simulink model "case6"  (R2024b)
settings: Solver=FixedStepAuto  StartTime=0  StopTime=1  FixedStep=1e-7  RelTol=1e-3
values from neighbouring files (symbols this model uses):
  SG_D_1_D = 0.01056    [IEEE9_case_parameters.m]    (also in case1_parameters.m; case2_parameters.m; case3_parameters.m; case4_parameters.m)
  SG_D_1_EnableSaturation = 0    [IEEE9_case_parameters.m]    (also in case1_parameters.m; case2_parameters.m; case3_parameters.m; case4_parameters.m)
  SG_D_1_f0 = 60    [IEEE9_case_parameters.m]    (also in case1_parameters.m; case2_parameters.m; case3_parameters.m; case4_parameters.m)
  SG_D_1_H = 7.5    [IEEE9_case_parameters.m]    (also in case1_parameters.m; case2_parameters.m; case3_parameters.m; case4_parameters.m)
  SG_D_1_K_A = 20    [IEEE9_case_parameters.m]    (also in case1_parameters.m; case2_parameters.m; case3_parameters.m; case4_parameters.m)
  SG_D_1_K_E = 1.000000e+1    (= 10)    [IEEE9_case_parameters.m]    (also in case1_parameters.m; case2_parameters.m; case3_parameters.m; case4_parameters.m)
  SG_D_1_K_F = 2.363    [IEEE9_case_parameters.m]    (also in case1_parameters.m; case2_parameters.m; case3_parameters.m; case4_parameters.m)
  SG_D_1_K_s = 0.5    [IEEE9_case_parameters.m]    (also in case1_parameters.m = 5; case2_parameters.m = 5; case3_parameters.m = 5; case4_parameters.m = 5)
  SG_D_1_R_a = 0.001088    [IEEE9_case_parameters.m]    (also in case1_parameters.m; case2_parameters.m; case3_parameters.m; case4_parameters.m)
  SG_D_1_S_A = 1    [IEEE9_case_parameters.m]    (also in case1_parameters.m; case2_parameters.m; case3_parameters.m; case4_parameters.m)
  SG_D_1_S_B = 0.103    [IEEE9_case_parameters.m]    (also in case1_parameters.m; case2_parameters.m; case3_parameters.m; case4_parameters.m)
  SG_D_1_S_N = 10.659857    [IEEE9_case_parameters.m]    (also in case1_parameters.m; case2_parameters.m; case3_parameters.m; case4_parameters.m)
  SG_D_1_SpeedPara = 200    [IEEE9_case_parameters.m]    (also in case1_parameters.m; case2_parameters.m; case3_parameters.m; case4_parameters.m)
  SG_D_1_T_0 = 0.720173    [IEEE9_case_parameters.m]    (also in case1_parameters.m = 0.755522; case2_parameters.m = 0.808931; case3_parameters.m = 0.869402; case4_parameters.m = 0.729316)
  SG_D_1_T_1 = 0.3    [IEEE9_case_parameters.m]    (also in case1_parameters.m; case2_parameters.m; case3_parameters.m; case4_parameters.m)
  SG_D_1_T_2 = 0.05    [IEEE9_case_parameters.m]    (also in case1_parameters.m; case2_parameters.m; case3_parameters.m; case4_parameters.m)
  SG_D_1_T_3 = 0.02    [IEEE9_case_parameters.m]    (also in case1_parameters.m; case2_parameters.m; case3_parameters.m; case4_parameters.m)
  SG_D_1_T_4 = 0.005    [IEEE9_case_parameters.m]    (also in case1_parameters.m; case2_parameters.m; case3_parameters.m; case4_parameters.m)
  SG_D_1_T_A = 0.02    [IEEE9_case_parameters.m]    (also in case1_parameters.m; case2_parameters.m; case3_parameters.m; case4_parameters.m)
  SG_D_1_T_dd = 8.000000e+0    (= 8)    [IEEE9_case_parameters.m]    (also in case1_parameters.m; case2_parameters.m; case3_parameters.m; case4_parameters.m)
  SG_D_1_T_ddd = 0.04    [IEEE9_case_parameters.m]    (also in case1_parameters.m; case2_parameters.m; case3_parameters.m; case4_parameters.m)
  SG_D_1_T_E = 0.314    [IEEE9_case_parameters.m]    (also in case1_parameters.m; case2_parameters.m; case3_parameters.m; case4_parameters.m)
  SG_D_1_T_F = 0.35    [IEEE9_case_parameters.m]    (also in case1_parameters.m; case2_parameters.m; case3_parameters.m; case4_parameters.m)
  SG_D_1_T_qd = 0.8    [IEEE9_case_parameters.m]    (also in case1_parameters.m; case2_parameters.m; case3_parameters.m; case4_parameters.m)
  SG_D_1_T_qdd = 0.02    [IEEE9_case_parameters.m]    (also in case1_parameters.m; case2_parameters.m; case3_parameters.m; case4_parameters.m)
  SG_D_1_T_speed = 0.1    [IEEE9_case_parameters.m]    (also in case1_parameters.m = 200; case2_parameters.m = 200; case3_parameters.m = 200; case4_parameters.m = 200)
  SG_D_1_T_w = 0.5    [IEEE9_case_parameters.m]    (also in case1_parameters.m; case2_parameters.m; case3_parameters.m; case4_parameters.m)
  SG_D_1_V_ref = 1.990276    [IEEE9_case_parameters.m]    (also in case1_parameters.m = 2.042296; case2_parameters.m = 2.051388; case3_parameters.m = 2.089584; case4_parameters.m = 2.01845)
  SG_D_1_w_ref = 376.991118    [IEEE9_case_parameters.m]    (also in case1_parameters.m; case2_parameters.m; case3_parameters.m; case4_parameters.m)
  SG_D_1_wb = 6.000000e+1    (= 60)    [IEEE9_case_parameters.m]    (also in case1_parameters.m; case2_parameters.m; case3_parameters.m; case4_parameters.m)
  SG_D_1_x_d = 1.9    [IEEE9_case_parameters.m]    (also in case1_parameters.m; case2_parameters.m; case3_parameters.m; case4_parameters.m)
  SG_D_1_x_dd = 0.302    [IEEE9_case_parameters.m]    (also in case1_parameters.m; case2_parameters.m; case3_parameters.m; case4_parameters.m)
  SG_D_1_x_ddd = 0.204    [IEEE9_case_parameters.m]    (also in case1_parameters.m; case2_parameters.m; case3_parameters.m; case4_parameters.m)
  SG_D_1_x_l = 0.05    [IEEE9_case_parameters.m]    (also in case1_parameters.m; case2_parameters.m; case3_parameters.m; case4_parameters.m)
  SG_D_1_x_q = 1.3    [IEEE9_case_parameters.m]    (also in case1_parameters.m; case2_parameters.m; case3_parameters.m; case4_parameters.m)
  SG_D_1_x_qd = 0.5    [IEEE9_case_parameters.m]    (also in case1_parameters.m; case2_parameters.m; case3_parameters.m; case4_parameters.m)
  SG_D_1_x_qdd = 0.3    [IEEE9_case_parameters.m]    (also in case1_parameters.m; case2_parameters.m; case3_parameters.m; case4_parameters.m)
  SG_D_2_D = 0.02    [IEEE9_case_parameters.m]    (also in case1_parameters.m; case2_parameters.m; case3_parameters.m; case4_parameters.m)
  SG_D_2_EnableSaturation = 0    [IEEE9_case_parameters.m]    (also in case1_parameters.m; case2_parameters.m; case3_parameters.m; case4_parameters.m)
  SG_D_2_f0 = 60    [IEEE9_case_parameters.m]    (also in case1_parameters.m; case2_parameters.m; case3_parameters.m; case4_parameters.m)
  SG_D_2_H = 8.000000e+0    (= 8)    [IEEE9_case_parameters.m]    (also in case1_parameters.m; case2_parameters.m; case3_parameters.m; case4_parameters.m)
  SG_D_2_K_A = 20    [IEEE9_case_parameters.m]    (also in case1_parameters.m; case2_parameters.m; case3_parameters.m; case4_parameters.m)
  SG_D_2_K_E = 1.000000e+1    (= 10)    [IEEE9_case_parameters.m]    (also in case1_parameters.m; case2_parameters.m; case3_parameters.m; case4_parameters.m)
  SG_D_2_K_F = 2.363    [IEEE9_case_parameters.m]    (also in case1_parameters.m; case2_parameters.m; case3_parameters.m; case4_parameters.m)
  SG_D_2_K_s = 0.5    [IEEE9_case_parameters.m]    (also in case1_parameters.m = 4; case2_parameters.m = 4; case3_parameters.m = 4; case4_parameters.m = 4)
  SG_D_2_R_a = 0.001088    [IEEE9_case_parameters.m]    (also in case1_parameters.m; case2_parameters.m; case3_parameters.m; case4_parameters.m)
  SG_D_2_S_A = 1    [IEEE9_case_parameters.m]    (also in case1_parameters.m; case2_parameters.m; case3_parameters.m; case4_parameters.m)
  SG_D_2_S_B = 0.103    [IEEE9_case_parameters.m]    (also in case1_parameters.m; case2_parameters.m; case3_parameters.m; case4_parameters.m)
  SG_D_2_S_N = 10.659857    [IEEE9_case_parameters.m]    (also in case1_parameters.m; case2_parameters.m; case3_parameters.m; case4_parameters.m)
  SG_D_2_SpeedPara = 200    [IEEE9_case_parameters.m]    (also in case1_parameters.m; case2_parameters.m; case3_parameters.m; case4_parameters.m)
  SG_D_2_T_0 = 1.632913    [IEEE9_case_parameters.m]    (also in case1_parameters.m = 1.632925; case2_parameters.m = 1.632915; case3_parameters.m = 1.632914; case4_parameters.m = 1.632927)
  SG_D_2_T_1 = 0.2    [IEEE9_case_parameters.m]    (also in case1_parameters.m; case2_parameters.m; case3_parameters.m; case4_parameters.m)
  SG_D_2_T_2 = 0.05    [IEEE9_case_parameters.m]    (also in case1_parameters.m; case2_parameters.m; case3_parameters.m; case4_parameters.m)
  SG_D_2_T_3 = 0.02    [IEEE9_case_parameters.m]    (also in case1_parameters.m; case2_parameters.m; case3_parameters.m; case4_parameters.m)
  SG_D_2_T_4 = 0.005    [IEEE9_case_parameters.m]    (also in case1_parameters.m; case2_parameters.m; case3_parameters.m; case4_parameters.m)
  SG_D_2_T_A = 0.02    [IEEE9_case_parameters.m]    (also in case1_parameters.m; case2_parameters.m; case3_parameters.m; case4_parameters.m)
  SG_D_2_T_dd = 7.9    [IEEE9_case_parameters.m]    (also in case1_parameters.m; case2_parameters.m; case3_parameters.m; case4_parameters.m)
  SG_D_2_T_ddd = 0.04    [IEEE9_case_parameters.m]    (also in case1_parameters.m; case2_parameters.m; case3_parameters.m; case4_parameters.m)
  SG_D_2_T_E = 0.314    [IEEE9_case_parameters.m]    (also in case1_parameters.m; case2_parameters.m; case3_parameters.m; case4_parameters.m)
  SG_D_2_T_F = 0.35    [IEEE9_case_parameters.m]    (also in case1_parameters.m; case2_parameters.m; case3_parameters.m; case4_parameters.m)
  SG_D_2_T_qd = 0.8    [IEEE9_case_parameters.m]    (also in case1_parameters.m; case2_parameters.m; case3_parameters.m; case4_parameters.m)
  SG_D_2_T_qdd = 0.015    [IEEE9_case_parameters.m]    (also in case1_parameters.m; case2_parameters.m; case3_parameters.m; case4_parameters.m)
  SG_D_2_T_speed = 0.1    [IEEE9_case_parameters.m]    (also in case1_parameters.m = 150; case2_parameters.m = 150; case3_parameters.m = 150; case4_parameters.m = 150)
  SG_D_2_T_w = 0.35    [IEEE9_case_parameters.m]    (also in case1_parameters.m; case2_parameters.m; case3_parameters.m; case4_parameters.m)
  SG_D_2_V_ref = 2.58547    [IEEE9_case_parameters.m]    (also in case1_parameters.m = 2.597896; case2_parameters.m = 2.587136; case3_parameters.m = 2.586042; case4_parameters.m = 2.599679)
  SG_D_2_w_ref = 376.991118    [IEEE9_case_parameters.m]    (also in case1_parameters.m; case2_parameters.m; case3_parameters.m; case4_parameters.m)
  SG_D_2_wb = 6.000000e+1    (= 60)    [IEEE9_case_parameters.m]    (also in case1_parameters.m; case2_parameters.m; case3_parameters.m; case4_parameters.m)
  SG_D_2_x_d = 1.8    [IEEE9_case_parameters.m]    (also in case1_parameters.m; case2_parameters.m; case3_parameters.m; case4_parameters.m)
  SG_D_2_x_dd = 0.302    [IEEE9_case_parameters.m]    (also in case1_parameters.m; case2_parameters.m; case3_parameters.m; case4_parameters.m)
  SG_D_2_x_ddd = 0.204    [IEEE9_case_parameters.m]    (also in case1_parameters.m; case2_parameters.m; case3_parameters.m; case4_parameters.m)
  SG_D_2_x_l = 0.05    [IEEE9_case_parameters.m]    (also in case1_parameters.m; case2_parameters.m; case3_parameters.m; case4_parameters.m)
  SG_D_2_x_q = 1.25    [IEEE9_case_parameters.m]    (also in case1_parameters.m; case2_parameters.m; case3_parameters.m; case4_parameters.m)
  SG_D_2_x_qd = 0.5    [IEEE9_case_parameters.m]    (also in case1_parameters.m; case2_parameters.m; case3_parameters.m; case4_parameters.m)
  SG_D_2_x_qdd = 0.3    [IEEE9_case_parameters.m]    (also in case1_parameters.m; case2_parameters.m; case3_parameters.m; case4_parameters.m)
  SG_D_3_D = 0.02    [IEEE9_case_parameters.m]    (also in case1_parameters.m; case2_parameters.m; case3_parameters.m; case4_parameters.m)
  SG_D_3_EnableSaturation = 0    [IEEE9_case_parameters.m]    (also in case1_parameters.m; case2_parameters.m; case3_parameters.m; case4_parameters.m)
  SG_D_3_f0 = 60    [IEEE9_case_parameters.m]    (also in case1_parameters.m; case2_parameters.m; case3_parameters.m; case4_parameters.m)
  SG_D_3_H = 7.7    [IEEE9_case_parameters.m]    (also in case1_parameters.m; case2_parameters.m; case3_parameters.m; case4_parameters.m)
  SG_D_3_K_A = 20    [IEEE9_case_parameters.m]    (also in case1_parameters.m; case2_parameters.m; case3_parameters.m; case4_parameters.m)
  SG_D_3_K_E = 1.000000e+1    (= 10)    [IEEE9_case_parameters.m]    (also in case1_parameters.m; case2_parameters.m; case3_parameters.m; case4_parameters.m)
  SG_D_3_K_F = 2.363    [IEEE9_case_parameters.m]    (also in case1_parameters.m; case2_parameters.m; case3_parameters.m; case4_parameters.m)
  SG_D_3_K_s = 0.2    [IEEE9_case_parameters.m]    (also in case1_parameters.m = 2; case2_parameters.m = 2; case3_parameters.m = 2; case4_parameters.m = 2)
  SG_D_3_R_a = 0.001088    [IEEE9_case_parameters.m]    (also in case1_parameters.m; case2_parameters.m; case3_parameters.m; case4_parameters.m)
  SG_D_3_S_A = 1    [IEEE9_case_parameters.m]    (also in case1_parameters.m; case2_parameters.m; case3_parameters.m; case4_parameters.m)
  SG_D_3_S_B = 0.103    [IEEE9_case_parameters.m]    (also in case1_parameters.m; case2_parameters.m; case3_parameters.m; case4_parameters.m)
  SG_D_3_S_N = 10.659857    [IEEE9_case_parameters.m]    (also in case1_parameters.m; case2_parameters.m; case3_parameters.m; case4_parameters.m)
  SG_D_3_SpeedPara = 200    [IEEE9_case_parameters.m]    (also in case1_parameters.m; case2_parameters.m; case3_parameters.m; case4_parameters.m)
  SG_D_3_T_0 = 0.850788    [IEEE9_case_parameters.m]    (also in case1_parameters.m = 0.850786; case2_parameters.m = 0.850787; case3_parameters.m; case4_parameters.m = 0.850786)
  SG_D_3_T_1 = 0.2    [IEEE9_case_parameters.m]    (also in case1_parameters.m; case2_parameters.m; case3_parameters.m; case4_parameters.m)
  SG_D_3_T_2 = 0.05    [IEEE9_case_parameters.m]    (also in case1_parameters.m; case2_parameters.m; case3_parameters.m; case4_parameters.m)
  SG_D_3_T_3 = 0.02    [IEEE9_case_parameters.m]    (also in case1_parameters.m; case2_parameters.m; case3_parameters.m; case4_parameters.m)
  SG_D_3_T_4 = 0.005    [IEEE9_case_parameters.m]    (also in case1_parameters.m; case2_parameters.m; case3_parameters.m; case4_parameters.m)
  SG_D_3_T_A = 0.02    [IEEE9_case_parameters.m]    (also in case1_parameters.m; case2_parameters.m; case3_parameters.m; case4_parameters.m)
  SG_D_3_T_dd = 8.1    [IEEE9_case_parameters.m]    (also in case1_parameters.m; case2_parameters.m; case3_parameters.m; case4_parameters.m)
  SG_D_3_T_ddd = 0.04    [IEEE9_case_parameters.m]    (also in case1_parameters.m; case2_parameters.m; case3_parameters.m; case4_parameters.m)
  SG_D_3_T_E = 0.314    [IEEE9_case_parameters.m]    (also in case1_parameters.m; case2_parameters.m; case3_parameters.m; case4_parameters.m)
  SG_D_3_T_F = 0.35    [IEEE9_case_parameters.m]    (also in case1_parameters.m; case2_parameters.m; case3_parameters.m; case4_parameters.m)
  SG_D_3_T_qd = 0.8    [IEEE9_case_parameters.m]    (also in case1_parameters.m; case2_parameters.m; case3_parameters.m; case4_parameters.m)
  SG_D_3_T_qdd = 0.015    [IEEE9_case_parameters.m]    (also in case1_parameters.m; case2_parameters.m; case3_parameters.m; case4_parameters.m)
  SG_D_3_T_speed = 0.1    [IEEE9_case_parameters.m]    (also in case1_parameters.m = 180; case2_parameters.m = 180; case3_parameters.m = 180; case4_parameters.m = 180)
  SG_D_3_T_w = 0.4    [IEEE9_case_parameters.m]    (also in case1_parameters.m; case2_parameters.m; case3_parameters.m; case4_parameters.m)
  SG_D_3_V_ref = 1.892727    [IEEE9_case_parameters.m]    (also in case1_parameters.m = 1.906439; case2_parameters.m = 1.895535; case3_parameters.m = 1.892105; case4_parameters.m = 1.906598)
  SG_D_3_w_ref = 376.991118    [IEEE9_case_parameters.m]    (also in case1_parameters.m; case2_parameters.m; case3_parameters.m; case4_parameters.m)
  SG_D_3_wb = 6.000000e+1    (= 60)    [IEEE9_case_parameters.m]    (also in case1_parameters.m; case2_parameters.m; case3_parameters.m; case4_parameters.m)
  SG_D_3_x_d = 1.85    [IEEE9_case_parameters.m]    (also in case1_parameters.m; case2_parameters.m; case3_parameters.m; case4_parameters.m)
  SG_D_3_x_dd = 0.302    [IEEE9_case_parameters.m]    (also in case1_parameters.m; case2_parameters.m; case3_parameters.m; case4_parameters.m)
  SG_D_3_x_ddd = 0.204    [IEEE9_case_parameters.m]    (also in case1_parameters.m; case2_parameters.m; case3_parameters.m; case4_parameters.m)
  SG_D_3_x_l = 0.05    [IEEE9_case_parameters.m]    (also in case1_parameters.m; case2_parameters.m; case3_parameters.m; case4_parameters.m)
  SG_D_3_x_q = 1.2    [IEEE9_case_parameters.m]    (also in case1_parameters.m; case2_parameters.m; case3_parameters.m; case4_parameters.m)
  SG_D_3_x_qd = 0.5    [IEEE9_case_parameters.m]    (also in case1_parameters.m; case2_parameters.m; case3_parameters.m; case4_parameters.m)
  SG_D_3_x_qdd = 0.3    [IEEE9_case_parameters.m]    (also in case1_parameters.m; case2_parameters.m; case3_parameters.m; case4_parameters.m)
(part 2 of 12)

== system case6/SG_D_2 ==
  v_d_SG_D_2 : Inport
  v_q_SG_D_2 : Inport  Port=2
  E_fd_SG_D_2 : Integrator  InitialCondition=3.1522779272193207
  Px_1_SG_D_2 : Integrator  InitialCondition=0.0
  Px_2_SG_D_2 : Integrator  InitialCondition=0.0
  Px_3_SG_D_2 : Integrator  InitialCondition=-2.786907381010745e-25
  R_f_SG_D_2 : Integrator  InitialCondition=21.28237926291216
  T_e_SG_D_2_block : Subsystem
  T_m_SG_D_2 : Integrator  InitialCondition=1.632905998125784
  V_f_SG_D_2 : Integrator  InitialCondition=31.52277927219321
  d_E_fd_SG_D_2_block : Subsystem
  d_Px_1_SG_D_2_block : Subsystem
  d_Px_2_SG_D_2_block : Subsystem
  d_Px_3_SG_D_2_block : Subsystem
  d_R_f_SG_D_2_block : Subsystem
  d_T_m_SG_D_2_block : Subsystem
  d_V_f_SG_D_2_block : Subsystem
  d_psi_1d_SG_D_2_block : Subsystem
  d_psi_d_SG_D_2_block : Subsystem
  d_psi_fd_SG_D_2_block : Subsystem
  d_psi_gq_SG_D_2_block : Subsystem
  d_psi_kq_SG_D_2_block : Subsystem
  d_psi_q_SG_D_2_block : Subsystem
  d_theta_SG_D_2_block : Subsystem
  d_w_SG_D_2_block : Subsystem
  i_d_SG_D_2_block : Subsystem
  i_q_SG_D_2_block : Subsystem
  psi_1d_SG_D_2 : Integrator  InitialCondition=0.5661877704992511
  psi_d_SG_D_2 : Integrator  InitialCondition=0.49229948030724896
  psi_fd_SG_D_2 : Integrator  InitialCondition=0.9385847530669411
  psi_gq_SG_D_2 : Integrator  InitialCondition=0.523477654580875
  psi_kq_SG_D_2 : Integrator  InitialCondition=-0.8375642473294
  psi_q_SG_D_2 : Integrator  InitialCondition=-0.8724627576347918
  theta_SG_D_2 : Integrator  InitialCondition=1.2302637808215569
  theta_SG_D_2_out_block : Subsystem
  w_SG_D_2 : Integrator  InitialCondition=376.99111843077515
  w_SG_D_2_out_block : Subsystem
  i_d_SG_D_2 : Outport
  i_q_SG_D_2 : Outport  Port=2
  T_e_SG_D_2 : Outport  Port=3
  w_SG_D_2_out : Outport  Port=4
  theta_SG_D_2_out : Outport  Port=5
  wires:
  T_e_SG_D_2_block/1(Blockout_T_e_SG_D_2_2a19a) -> T_e_SG_D_2/1
  d_Px_2_SG_D_2_block/1(Blockout_d_Px_2_SG_D_2_75597) -> Px_2_SG_D_2/1
  d_T_m_SG_D_2_block/1(Blockout_d_T_m_SG_D_2_8c4dc) -> T_m_SG_D_2/1
  w_SG_D_2/1 -> d_psi_d_SG_D_2_block/9(State_w_SG_D_2_32109), d_w_SG_D_2_block/1(State_w_SG_D_2_9540e), d_psi_q_SG_D_2_block/9(State_w_SG_D_2_3c58c), d_V_f_SG_D_2_block/8(State_w_SG_D_2_9ec77), d_V_f_SG_D_2_block/13(State_w_SG_D_2_fc7ef), d_theta_SG_D_2_block/1(State_w_SG_D_2_cb344), d_Px_1_SG_D_2_block/2(State_w_SG_D_2_e2895), d_T_m_SG_D_2_block/1(State_w_SG_D_2_d1516), d_Px_2_SG_D_2_block/4(State_w_SG_D_2_c3292), w_SG_D_2_out_block/1(State_w_SG_D_2_a7da0), d_Px_3_SG_D_2_block/6(State_w_SG_D_2_e2d04)
  psi_q_SG_D_2/1 -> d_psi_d_SG_D_2_block/8(State_psi_q_SG_D_2_e45e5), d_psi_gq_SG_D_2_block/6(State_psi_q_SG_D_2_3086c), d_psi_kq_SG_D_2_block/5(State_psi_q_SG_D_2_b3f78), d_w_SG_D_2_block/6(State_psi_q_SG_D_2_7f967), d_w_SG_D_2_block/7(State_psi_q_SG_D_2_af0e3), d_V_f_SG_D_2_block/11(State_psi_q_SG_D_2_aa693), d_psi_q_SG_D_2_block/3(State_psi_q_SG_D_2_571db), i_d_SG_D_2_block/3(State_psi_q_SG_D_2_46eac), T_e_SG_D_2_block/4(State_psi_q_SG_D_2_aa98c), d_psi_gq_SG_D_2_block/9(State_psi_q_SG_D_2_9e01f), T_e_SG_D_2_block/5(State_psi_q_SG_D_2_0c973), i_q_SG_D_2_block/3(State_psi_q_SG_D_2_e3c89), d_V_f_SG_D_2_block/7(State_psi_q_SG_D_2_f03d5)
  w_SG_D_2_out_block/1(Blockout_w_SG_D_2_out_1bf45) -> w_SG_D_2_out/1
  d_theta_SG_D_2_block/1(Blockout_d_theta_SG_D_2_0f7ec) -> theta_SG_D_2/1
  psi_kq_SG_D_2/1 -> d_psi_q_SG_D_2_block/2(State_psi_kq_SG_D_2_25a64), d_psi_gq_SG_D_2_block/3(State_psi_kq_SG_D_2_00780), d_psi_gq_SG_D_2_block/5(State_psi_kq_SG_D_2_d1b3d), d_psi_kq_SG_D_2_block/2(State_psi_kq_SG_D_2_17791), d_w_SG_D_2_block/5(State_psi_kq_SG_D_2_8152c), d_V_f_SG_D_2_block/10(State_psi_kq_SG_D_2_e2d6f), d_psi_gq_SG_D_2_block/8(State_psi_kq_SG_D_2_4b899), i_d_SG_D_2_block/2(State_psi_kq_SG_D_2_f39d8), d_psi_kq_SG_D_2_block/4(State_psi_kq_SG_D_2_51ab3), i_q_SG_D_2_block/2(State_psi_kq_SG_D_2_930b2), T_e_SG_D_2_block/3(State_psi_kq_SG_D_2_bf31f)
  d_Px_1_SG_D_2_block/1(Blockout_d_Px_1_SG_D_2_cd7c4) -> Px_1_SG_D_2/1
  d_Px_3_SG_D_2_block/1(Blockout_d_Px_3_SG_D_2_4fae6) -> Px_3_SG_D_2/1
  T_m_SG_D_2/1 -> d_T_m_SG_D_2_block/2(State_T_m_SG_D_2_36b08), d_w_SG_D_2_block/2(State_T_m_SG_D_2_05bd7)
  Px_2_SG_D_2/1 -> d_Px_3_SG_D_2_block/2(State_Px_2_SG_D_2_d06b1), d_Px_2_SG_D_2_block/1(State_Px_2_SG_D_2_b5883), d_Px_3_SG_D_2_block/3(State_Px_2_SG_D_2_72320)
  i_d_SG_D_2_block/1(Blockout_i_d_SG_D_2_1c8b0) -> i_d_SG_D_2/1
  psi_d_SG_D_2/1 -> d_psi_fd_SG_D_2_block/6(State_psi_d_SG_D_2_52887), d_psi_fd_SG_D_2_block/9(State_psi_d_SG_D_2_9b3b0), d_psi_d_SG_D_2_block/2(State_psi_d_SG_D_2_1074f), d_psi_q_SG_D_2_block/8(State_psi_d_SG_D_2_57873), d_psi_1d_SG_D_2_block/4(State_psi_d_SG_D_2_2211c), d_w_SG_D_2_block/3(State_psi_d_SG_D_2_9dc7c), d_V_f_SG_D_2_block/5(State_psi_d_SG_D_2_4bbd3), d_V_f_SG_D_2_block/12(State_psi_d_SG_D_2_77c88), i_d_SG_D_2_block/6(State_psi_d_SG_D_2_503d3), T_e_SG_D_2_block/1(State_psi_d_SG_D_2_01b1a), i_q_SG_D_2_block/6(State_psi_d_SG_D_2_f3333), d_w_SG_D_2_block/9(State_psi_d_SG_D_2_75c16), T_e_SG_D_2_block/7(State_psi_d_SG_D_2_d0b7a)
  Px_1_SG_D_2/1 -> d_Px_2_SG_D_2_block/3(State_Px_1_SG_D_2_e0226), d_Px_3_SG_D_2_block/5(State_Px_1_SG_D_2_c353d), d_Px_3_SG_D_2_block/4(State_Px_1_SG_D_2_bdfda), d_Px_1_SG_D_2_block/1(State_Px_1_SG_D_2_84b2f), d_Px_2_SG_D_2_block/2(State_Px_1_SG_D_2_b4148)
  psi_gq_SG_D_2/1 -> d_psi_q_SG_D_2_block/1(State_psi_gq_SG_D_2_12de1), d_psi_gq_SG_D_2_block/1(State_psi_gq_SG_D_2_36994), d_psi_gq_SG_D_2_block/2(State_psi_gq_SG_D_2_8aea1), d_psi_gq_SG_D_2_block/4(State_psi_gq_SG_D_2_0cdbf), d_psi_kq_SG_D_2_block/1(State_psi_gq_SG_D_2_dc43a), d_w_SG_D_2_block/4(State_psi_gq_SG_D_2_1ea7a), d_psi_gq_SG_D_2_block/7(State_psi_gq_SG_D_2_14d3b), i_d_SG_D_2_block/1(State_psi_gq_SG_D_2_4eb5b), i_q_SG_D_2_block/1(State_psi_gq_SG_D_2_a612b), d_V_f_SG_D_2_block/9(State_psi_gq_SG_D_2_3a559), T_e_SG_D_2_block/2(State_psi_gq_SG_D_2_1bd12), d_psi_kq_SG_D_2_block/3(State_psi_gq_SG_D_2_a7d32)
  v_d_SG_D_2/1 -> d_psi_d_SG_D_2_block/4(Input_v_d_SG_D_2_2f023), d_psi_q_SG_D_2_block/4(Input_v_d_SG_D_2_48357)
  d_V_f_SG_D_2_block/1(Blockout_d_V_f_SG_D_2_54ac8) -> V_f_SG_D_2/1
  v_q_SG_D_2/1 -> d_psi_d_SG_D_2_block/6(Input_v_q_SG_D_2_18101), d_psi_q_SG_D_2_block/6(Input_v_q_SG_D_2_9b22c)
  theta_SG_D_2/1 -> d_psi_d_SG_D_2_block/5(State_theta_SG_D_2_812e2), d_psi_d_SG_D_2_block/7(State_theta_SG_D_2_15477), d_psi_q_SG_D_2_block/5(State_theta_SG_D_2_b5a9c), i_d_SG_D_2_block/4(State_theta_SG_D_2_9c587), i_d_SG_D_2_block/8(State_theta_SG_D_2_8a3e8), d_psi_q_SG_D_2_block/7(State_theta_SG_D_2_25188), i_q_SG_D_2_block/8(State_theta_SG_D_2_4cc38), theta_SG_D_2_out_block/1(State_theta_SG_D_2_6ea16), i_q_SG_D_2_block/4(State_theta_SG_D_2_df516)
  psi_1d_SG_D_2/1 -> d_psi_fd_SG_D_2_block/3(State_psi_1d_SG_D_2_6d215), d_psi_fd_SG_D_2_block/5(State_psi_1d_SG_D_2_0a0a1), d_psi_fd_SG_D_2_block/8(State_psi_1d_SG_D_2_47eb6), d_psi_d_SG_D_2_block/1(State_psi_1d_SG_D_2_35cf0), d_psi_1d_SG_D_2_block/1(State_psi_1d_SG_D_2_5b9a9), d_V_f_SG_D_2_block/4(State_psi_1d_SG_D_2_d8f0b), d_w_SG_D_2_block/8(State_psi_1d_SG_D_2_c88b6), i_q_SG_D_2_block/5(State_psi_1d_SG_D_2_ac141), T_e_SG_D_2_block/6(State_psi_1d_SG_D_2_e8fde), d_psi_1d_SG_D_2_block/3(State_psi_1d_SG_D_2_2957b), i_d_SG_D_2_block/5(State_psi_1d_SG_D_2_487b1)
  psi_fd_SG_D_2/1 -> d_psi_fd_SG_D_2_block/4(State_psi_fd_SG_D_2_241bb), d_psi_fd_SG_D_2_block/7(State_psi_fd_SG_D_2_e38e9), d_psi_fd_SG_D_2_block/10(State_psi_fd_SG_D_2_b670f), d_psi_fd_SG_D_2_block/2(State_psi_fd_SG_D_2_303fb), d_psi_d_SG_D_2_block/3(State_psi_fd_SG_D_2_72eef), d_w_SG_D_2_block/10(State_psi_fd_SG_D_2_33fe8), d_V_f_SG_D_2_block/6(State_psi_fd_SG_D_2_76e98), i_d_SG_D_2_block/7(State_psi_fd_SG_D_2_72c98), d_psi_1d_SG_D_2_block/2(State_psi_fd_SG_D_2_5c5ab), i_q_SG_D_2_block/7(State_psi_fd_SG_D_2_0104a), T_e_SG_D_2_block/8(State_psi_fd_SG_D_2_ce60b), d_psi_1d_SG_D_2_block/5(State_psi_fd_SG_D_2_68d1a)
  d_R_f_SG_D_2_block/1(Blockout_d_R_f_SG_D_2_cc0fa) -> R_f_SG_D_2/1
  d_psi_kq_SG_D_2_block/1(Blockout_d_psi_kq_SG_D_2_04077) -> psi_kq_SG_D_2/1
  d_w_SG_D_2_block/1(Blockout_d_w_SG_D_2_78019) -> w_SG_D_2/1
  d_psi_gq_SG_D_2_block/1(Blockout_d_psi_gq_SG_D_2_441f6) -> psi_gq_SG_D_2/1
  d_psi_q_SG_D_2_block/1(Blockout_d_psi_q_SG_D_2_fdda2) -> psi_q_SG_D_2/1
  i_q_SG_D_2_block/1(Blockout_i_q_SG_D_2_fe66f) -> i_q_SG_D_2/1
  d_psi_d_SG_D_2_block/1(Blockout_d_psi_d_SG_D_2_5e9d3) -> psi_d_SG_D_2/1
  R_f_SG_D_2/1 -> d_R_f_SG_D_2_block/2(State_R_f_SG_D_2_02ca4), d_V_f_SG_D_2_block/2(State_R_f_SG_D_2_5f724)
  theta_SG_D_2_out_block/1(Blockout_theta_SG_D_2_out_19715) -> theta_SG_D_2_out/1
  d_psi_1d_SG_D_2_block/1(Blockout_d_psi_1d_SG_D_2_a3cd5) -> psi_1d_SG_D_2/1
  V_f_SG_D_2/1 -> d_V_f_SG_D_2_block/14(State_V_f_SG_D_2_9b9ce), d_E_fd_SG_D_2_block/2(State_V_f_SG_D_2_6a733)
  Px_3_SG_D_2/1 -> d_V_f_SG_D_2_block/3(State_Px_3_SG_D_2_19ed3), d_Px_3_SG_D_2_block/1(State_Px_3_SG_D_2_5e818)
  d_E_fd_SG_D_2_block/1(Blockout_d_E_fd_SG_D_2_9f684) -> E_fd_SG_D_2/1
  E_fd_SG_D_2/1 -> d_V_f_SG_D_2_block/1(State_E_fd_SG_D_2_3ccac), d_R_f_SG_D_2_block/1(State_E_fd_SG_D_2_5e385), d_E_fd_SG_D_2_block/1(State_E_fd_SG_D_2_81070), d_psi_fd_SG_D_2_block/1(State_E_fd_SG_D_2_19eb9)
  d_psi_fd_SG_D_2_block/1(Blockout_d_psi_fd_SG_D_2_3f1a9) -> psi_fd_SG_D_2/1

== system case6/SG_D_3 ==
  v_d_SG_D_3 : Inport
  v_q_SG_D_3 : Inport  Port=2
  E_fd_SG_D_3 : Integrator  InitialCondition=1.770368251781124
  Px_1_SG_D_3 : Integrator  InitialCondition=0.0
  Px_2_SG_D_3 : Integrator  InitialCondition=0.0
  Px_3_SG_D_3 : Integrator  InitialCondition=8.67782857201044e-25
  R_f_SG_D_3 : Integrator  InitialCondition=11.952514797025131
  T_e_SG_D_3_block : Subsystem
  T_m_SG_D_3 : Integrator  InitialCondition=0.8507889607782718
  V_f_SG_D_3 : Integrator  InitialCondition=17.70368251781124
  d_E_fd_SG_D_3_block : Subsystem
  d_Px_1_SG_D_3_block : Subsystem
  d_Px_2_SG_D_3_block : Subsystem
  d_Px_3_SG_D_3_block : Subsystem
  d_R_f_SG_D_3_block : Subsystem
  d_T_m_SG_D_3_block : Subsystem
  d_V_f_SG_D_3_block : Subsystem
  d_psi_1d_SG_D_3_block : Subsystem
  d_psi_d_SG_D_3_block : Subsystem
  d_psi_fd_SG_D_3_block : Subsystem
  d_psi_gq_SG_D_3_block : Subsystem
  d_psi_kq_SG_D_3_block : Subsystem
  d_psi_q_SG_D_3_block : Subsystem
  d_theta_SG_D_3_block : Subsystem
  d_w_SG_D_3_block : Subsystem
  i_d_SG_D_3_block : Subsystem
  i_q_SG_D_3_block : Subsystem
  psi_1d_SG_D_3 : Integrator  InitialCondition=0.7075299759323115
  psi_d_SG_D_3 : Integrator  InitialCondition=0.6780066904920665
  psi_fd_SG_D_3 : Integrator  InitialCondition=0.8563273345511452
  psi_gq_SG_D_3 : Integrator  InitialCondition=0.4295161353431842
  psi_kq_SG_D_3 : Integrator  InitialCondition=-0.7056336509209455
  psi_q_SG_D_3 : Integrator  InitialCondition=-0.7363133748740301
  theta_SG_D_3 : Integrator  InitialCondition=0.9182325005313983
  theta_SG_D_3_out_block : Subsystem
  w_SG_D_3 : Integrator  InitialCondition=376.99111843077515
  w_SG_D_3_out_block : Subsystem
  i_d_SG_D_3 : Outport
  i_q_SG_D_3 : Outport  Port=2
  T_e_SG_D_3 : Outport  Port=3
  w_SG_D_3_out : Outport  Port=4
  theta_SG_D_3_out : Outport  Port=5
  wires:
  d_Px_1_SG_D_3_block/1(Blockout_d_Px_1_SG_D_3_53c6c) -> Px_1_SG_D_3/1
  w_SG_D_3/1 -> d_V_f_SG_D_3_block/13(State_w_SG_D_3_7d0cc), d_psi_d_SG_D_3_block/9(State_w_SG_D_3_524fa), d_psi_q_SG_D_3_block/9(State_w_SG_D_3_8c018), d_V_f_SG_D_3_block/8(State_w_SG_D_3_12008), d_T_m_SG_D_3_block/1(State_w_SG_D_3_7ff4f), d_Px_1_SG_D_3_block/2(State_w_SG_D_3_9d504), d_Px_2_SG_D_3_block/4(State_w_SG_D_3_d4530), d_Px_3_SG_D_3_block/6(State_w_SG_D_3_25f91), d_w_SG_D_3_block/1(State_w_SG_D_3_b64e9), d_theta_SG_D_3_block/1(State_w_SG_D_3_8bed8), w_SG_D_3_out_block/1(State_w_SG_D_3_5dfed)
  d_T_m_SG_D_3_block/1(Blockout_d_T_m_SG_D_3_a2b29) -> T_m_SG_D_3/1
  R_f_SG_D_3/1 -> d_R_f_SG_D_3_block/2(State_R_f_SG_D_3_894c1), d_V_f_SG_D_3_block/2(State_R_f_SG_D_3_ab293)
  w_SG_D_3_out_block/1(Blockout_w_SG_D_3_out_62c16) -> w_SG_D_3_out/1
  d_Px_2_SG_D_3_block/1(Blockout_d_Px_2_SG_D_3_5e411) -> Px_2_SG_D_3/1
  d_w_SG_D_3_block/1(Blockout_d_w_SG_D_3_42d82) -> w_SG_D_3/1
  Px_1_SG_D_3/1 -> d_Px_2_SG_D_3_block/3(State_Px_1_SG_D_3_990a4), d_Px_3_SG_D_3_block/4(State_Px_1_SG_D_3_51d69), d_Px_2_SG_D_3_block/2(State_Px_1_SG_D_3_3f3ed), d_Px_3_SG_D_3_block/5(State_Px_1_SG_D_3_84b56), d_Px_1_SG_D_3_block/1(State_Px_1_SG_D_3_e4615)
  d_theta_SG_D_3_block/1(Blockout_d_theta_SG_D_3_22a58) -> theta_SG_D_3/1
  psi_fd_SG_D_3/1 -> d_psi_fd_SG_D_3_block/4(State_psi_fd_SG_D_3_e6b96), d_psi_fd_SG_D_3_block/10(State_psi_fd_SG_D_3_adc17), d_psi_fd_SG_D_3_block/2(State_psi_fd_SG_D_3_bb77c), d_psi_fd_SG_D_3_block/7(State_psi_fd_SG_D_3_c3c1b), d_psi_d_SG_D_3_block/3(State_psi_fd_SG_D_3_948b2), d_psi_1d_SG_D_3_block/2(State_psi_fd_SG_D_3_60e66), d_psi_1d_SG_D_3_block/5(State_psi_fd_SG_D_3_e1029), d_V_f_SG_D_3_block/6(State_psi_fd_SG_D_3_06b43), i_q_SG_D_3_block/7(State_psi_fd_SG_D_3_10fac), d_w_SG_D_3_block/10(State_psi_fd_SG_D_3_99630), T_e_SG_D_3_block/8(State_psi_fd_SG_D_3_9ec58), i_d_SG_D_3_block/7(State_psi_fd_SG_D_3_236ec)
  d_Px_3_SG_D_3_block/1(Blockout_d_Px_3_SG_D_3_ed081) -> Px_3_SG_D_3/1
  T_m_SG_D_3/1 -> d_T_m_SG_D_3_block/2(State_T_m_SG_D_3_3eb97), d_w_SG_D_3_block/2(State_T_m_SG_D_3_06ec9)
  v_d_SG_D_3/1 -> d_psi_d_SG_D_3_block/4(Input_v_d_SG_D_3_f4246), d_psi_q_SG_D_3_block/4(Input_v_d_SG_D_3_e9461)
  v_q_SG_D_3/1 -> d_psi_d_SG_D_3_block/6(Input_v_q_SG_D_3_8b8d5), d_psi_q_SG_D_3_block/6(Input_v_q_SG_D_3_d5a90)
  psi_q_SG_D_3/1 -> d_psi_d_SG_D_3_block/8(State_psi_q_SG_D_3_688d6), d_psi_q_SG_D_3_block/3(State_psi_q_SG_D_3_3f014), d_psi_gq_SG_D_3_block/9(State_psi_q_SG_D_3_aa05a), d_psi_kq_SG_D_3_block/5(State_psi_q_SG_D_3_2ea7c), d_V_f_SG_D_3_block/11(State_psi_q_SG_D_3_d993e), i_d_SG_D_3_block/3(State_psi_q_SG_D_3_eb21b), d_w_SG_D_3_block/7(State_psi_q_SG_D_3_a63b1), d_psi_gq_SG_D_3_block/6(State_psi_q_SG_D_3_03b15), d_V_f_SG_D_3_block/7(State_psi_q_SG_D_3_eff21), T_e_SG_D_3_block/4(State_psi_q_SG_D_3_17496), d_w_SG_D_3_block/6(State_psi_q_SG_D_3_29a7f), i_q_SG_D_3_block/3(State_psi_q_SG_D_3_c7c55), T_e_SG_D_3_block/5(State_psi_q_SG_D_3_1f719)
  Px_2_SG_D_3/1 -> d_Px_2_SG_D_3_block/1(State_Px_2_SG_D_3_c51e0), d_Px_3_SG_D_3_block/2(State_Px_2_SG_D_3_9ab37), d_Px_3_SG_D_3_block/3(State_Px_2_SG_D_3_8a812)
  psi_gq_SG_D_3/1 -> d_psi_q_SG_D_3_block/1(State_psi_gq_SG_D_3_44472), d_psi_gq_SG_D_3_block/1(State_psi_gq_SG_D_3_447cf), d_psi_gq_SG_D_3_block/2(State_psi_gq_SG_D_3_c8279), d_psi_gq_SG_D_3_block/4(State_psi_gq_SG_D_3_c97d9), d_psi_kq_SG_D_3_block/1(State_psi_gq_SG_D_3_3c968), d_V_f_SG_D_3_block/9(State_psi_gq_SG_D_3_4c437), i_d_SG_D_3_block/1(State_psi_gq_SG_D_3_f8709), d_w_SG_D_3_block/4(State_psi_gq_SG_D_3_0465b), i_q_SG_D_3_block/1(State_psi_gq_SG_D_3_2bc6a), d_psi_kq_SG_D_3_block/3(State_psi_gq_SG_D_3_f59cb), d_psi_gq_SG_D_3_block/7(State_psi_gq_SG_D_3_1930f), T_e_SG_D_3_block/2(State_psi_gq_SG_D_3_0552d)
  psi_kq_SG_D_3/1 -> d_psi_gq_SG_D_3_block/3(State_psi_kq_SG_D_3_7c168), d_psi_kq_SG_D_3_block/2(State_psi_kq_SG_D_3_3550c), d_psi_kq_SG_D_3_block/4(State_psi_kq_SG_D_3_48ef7), d_w_SG_D_3_block/5(State_psi_kq_SG_D_3_af6b0), d_psi_q_SG_D_3_block/2(State_psi_kq_SG_D_3_a31f2), i_d_SG_D_3_block/2(State_psi_kq_SG_D_3_4574d), d_V_f_SG_D_3_block/10(State_psi_kq_SG_D_3_cf6d4), i_q_SG_D_3_block/2(State_psi_kq_SG_D_3_393d8), T_e_SG_D_3_block/3(State_psi_kq_SG_D_3_0f4bf), d_psi_gq_SG_D_3_block/5(State_psi_kq_SG_D_3_d5a6f), d_psi_gq_SG_D_3_block/8(State_psi_kq_SG_D_3_5450f)
  d_psi_kq_SG_D_3_block/1(Blockout_d_psi_kq_SG_D_3_6fe0f) -> psi_kq_SG_D_3/1
  psi_1d_SG_D_3/1 -> d_psi_fd_SG_D_3_block/3(State_psi_1d_SG_D_3_acd54), d_psi_fd_SG_D_3_block/5(State_psi_1d_SG_D_3_a7b03), d_psi_fd_SG_D_3_block/8(State_psi_1d_SG_D_3_8d0f1), d_psi_d_SG_D_3_block/1(State_psi_1d_SG_D_3_bf921), d_psi_1d_SG_D_3_block/1(State_psi_1d_SG_D_3_8c5b0), d_w_SG_D_3_block/8(State_psi_1d_SG_D_3_34275), d_V_f_SG_D_3_block/4(State_psi_1d_SG_D_3_69975), i_d_SG_D_3_block/5(State_psi_1d_SG_D_3_699bf), i_q_SG_D_3_block/5(State_psi_1d_SG_D_3_724b9), d_psi_1d_SG_D_3_block/3(State_psi_1d_SG_D_3_8d87a), T_e_SG_D_3_block/6(State_psi_1d_SG_D_3_b9c0b)
  theta_SG_D_3/1 -> d_psi_d_SG_D_3_block/5(State_theta_SG_D_3_420f3), d_psi_d_SG_D_3_block/7(State_theta_SG_D_3_6650a), i_d_SG_D_3_block/4(State_theta_SG_D_3_5e6c6), i_q_SG_D_3_block/4(State_theta_SG_D_3_1e6e2), i_q_SG_D_3_block/8(State_theta_SG_D_3_90406), d_psi_q_SG_D_3_block/7(State_theta_SG_D_3_e3679), i_d_SG_D_3_block/8(State_theta_SG_D_3_8c3e3), d_psi_q_SG_D_3_block/5(State_theta_SG_D_3_3efc2), theta_SG_D_3_out_block/1(State_theta_SG_D_3_add6c)
  psi_d_SG_D_3/1 -> d_psi_fd_SG_D_3_block/6(State_psi_d_SG_D_3_c1f6f), d_psi_fd_SG_D_3_block/9(State_psi_d_SG_D_3_aa4bd), d_psi_d_SG_D_3_block/2(State_psi_d_SG_D_3_ef1bf), d_psi_q_SG_D_3_block/8(State_psi_d_SG_D_3_960b3), d_w_SG_D_3_block/9(State_psi_d_SG_D_3_ebe1b), d_w_SG_D_3_block/3(State_psi_d_SG_D_3_ca8ee), d_V_f_SG_D_3_block/12(State_psi_d_SG_D_3_44652), i_d_SG_D_3_block/6(State_psi_d_SG_D_3_b37a4), i_q_SG_D_3_block/6(State_psi_d_SG_D_3_a517e), T_e_SG_D_3_block/1(State_psi_d_SG_D_3_8bdd5), T_e_SG_D_3_block/7(State_psi_d_SG_D_3_c2826), d_V_f_SG_D_3_block/5(State_psi_d_SG_D_3_492f8), d_psi_1d_SG_D_3_block/4(State_psi_d_SG_D_3_b075c)
  d_R_f_SG_D_3_block/1(Blockout_d_R_f_SG_D_3_3e157) -> R_f_SG_D_3/1
  d_psi_q_SG_D_3_block/1(Blockout_d_psi_q_SG_D_3_c3e35) -> psi_q_SG_D_3/1
  T_e_SG_D_3_block/1(Blockout_T_e_SG_D_3_697bf) -> T_e_SG_D_3/1
  theta_SG_D_3_out_block/1(Blockout_theta_SG_D_3_out_34478) -> theta_SG_D_3_out/1
  d_V_f_SG_D_3_block/1(Blockout_d_V_f_SG_D_3_70847) -> V_f_SG_D_3/1
  d_psi_1d_SG_D_3_block/1(Blockout_d_psi_1d_SG_D_3_f8e09) -> psi_1d_SG_D_3/1
  d_psi_gq_SG_D_3_block/1(Blockout_d_psi_gq_SG_D_3_2ad5d) -> psi_gq_SG_D_3/1
  i_d_SG_D_3_block/1(Blockout_i_d_SG_D_3_01a92) -> i_d_SG_D_3/1
  d_psi_d_SG_D_3_block/1(Blockout_d_psi_d_SG_D_3_19103) -> psi_d_SG_D_3/1
  i_q_SG_D_3_block/1(Blockout_i_q_SG_D_3_27306) -> i_q_SG_D_3/1
  V_f_SG_D_3/1 -> d_V_f_SG_D_3_block/14(State_V_f_SG_D_3_1df36), d_E_fd_SG_D_3_block/2(State_V_f_SG_D_3_e8ba7)
  Px_3_SG_D_3/1 -> d_V_f_SG_D_3_block/3(State_Px_3_SG_D_3_58129), d_Px_3_SG_D_3_block/1(State_Px_3_SG_D_3_009d1)
  d_E_fd_SG_D_3_block/1(Blockout_d_E_fd_SG_D_3_557e1) -> E_fd_SG_D_3/1
  E_fd_SG_D_3/1 -> d_V_f_SG_D_3_block/1(State_E_fd_SG_D_3_edb23), d_R_f_SG_D_3_block/1(State_E_fd_SG_D_3_171e0), d_E_fd_SG_D_3_block/1(State_E_fd_SG_D_3_b4832), d_psi_fd_SG_D_3_block/1(State_E_fd_SG_D_3_340a0)
  d_psi_fd_SG_D_3_block/1(Blockout_d_psi_fd_SG_D_3_d3b7a) -> psi_fd_SG_D_3/1

== system case6/AC_1/d_id_line_1_4_block ==
  note: d_id_line_1_4 in case6
      | $376.991118430775\,\mathrm{iq}_{\mathrm{line},1,4}+6868.34433494245\,\mathrm{vd}_{\mathrm{bus},1}-6868.34433494245\,\mathrm{vd}_{\mathrm{bus},4}$
      | Automatically generated on 2025-10-31 19:20:47 .
  State_iq_line_1_4_12ad7 : Inport
  State_vd_bus_1_ef6b0 : Inport  Port=2
  State_vd_bus_4_e5c5f : Inport  Port=3
  Add_6d8e0 : Sum
  Constant_376.991118430775_47db6 : Constant  Value=376.991118430775
  Constant_6868.34433494245_03add : Constant  Value=6868.34433494245
  Constant_6868.34433494245_980d0 : Constant  Value=6868.34433494245
  Product_33cbf : Product
  Product_5c8fb : Product
  Product_d09b7 : Product
  Subtract_fa3b1 : Sum  Inputs=+-
  Blockout_d_id_line_1_4_9b681 : Outport
  wires:
  Constant_376.991118430775_47db6/1 -> Product_5c8fb/1
  Product_d09b7/1 -> Add_6d8e0/2
  State_iq_line_1_4_12ad7/1 -> Product_5c8fb/2
  Subtract_fa3b1/1 -> Blockout_d_id_line_1_4_9b681/1
  Constant_6868.34433494245_03add/1 -> Product_d09b7/1
  Product_5c8fb/1 -> Add_6d8e0/1
  State_vd_bus_1_ef6b0/1 -> Product_d09b7/2
  Constant_6868.34433494245_980d0/1 -> Product_33cbf/1
  State_vd_bus_4_e5c5f/1 -> Product_33cbf/2
  Add_6d8e0/1 -> Subtract_fa3b1/1
  Product_33cbf/1 -> Subtract_fa3b1/2

== system case6/AC_1/d_id_line_3_6_block ==
  note: d_id_line_3_6 in case6
      | $376.991118430775\,\mathrm{iq}_{\mathrm{line},3,6}+6751.13709373183\,\mathrm{vd}_{\mathrm{bus},3}-6751.13709373183\,\mathrm{vd}_{\mathrm{bus},6}$
      | Automatically generated on 2025-10-31 19:20:56 .
  State_iq_line_3_6_1fda9 : Inport
  State_vd_bus_3_b5b7a : Inport  Port=2
  State_vd_bus_6_77dc2 : Inport  Port=3
  Add_0d8a9 : Sum
  Constant_376.991118430775_69b36 : Constant  Value=376.991118430775
  Constant_6751.13709373183_86ee7 : Constant  Value=6751.13709373183
  Constant_6751.13709373183_c0697 : Constant  Value=6751.13709373183
  Product_49f41 : Product
  Product_6a75f : Product
  Product_bccce : Product
  Subtract_d28cb : Sum  Inputs=+-
  Blockout_d_id_line_3_6_6537b : Outport
  wires:
  State_vd_bus_3_b5b7a/1 -> Product_49f41/2
  Constant_376.991118430775_69b36/1 -> Product_bccce/1
  Product_49f41/1 -> Add_0d8a9/2
  State_iq_line_3_6_1fda9/1 -> Product_bccce/2
  Constant_6751.13709373183_c0697/1 -> Product_49f41/1
  Product_bccce/1 -> Add_0d8a9/1
  Constant_6751.13709373183_86ee7/1 -> Product_6a75f/1
  State_vd_bus_6_77dc2/1 -> Product_6a75f/2
  Add_0d8a9/1 -> Subtract_d28cb/1
  Product_6a75f/1 -> Subtract_d28cb/2
  Subtract_d28cb/1 -> Blockout_d_id_line_3_6_6537b/1

== system case6/AC_1/d_id_line_4_5_block ==
  note: d_id_line_4_5 in case6
      | $376.991118430775\,\mathrm{iq}_{\mathrm{line},4,5}-80.0510363901558\,\mathrm{id}_{\mathrm{line},4,5}+4300.18080100745\,\mathrm{vd}_{\mathrm{bus},4}-4300.18080100745\,\mathrm{vd}_{\mathrm{bus},5}$
      | Automatically generated on 2025-10-31 19:20:50 .
  State_id_line_4_5_ad13b : Inport
  State_iq_line_4_5_080ac : Inport  Port=2
  State_vd_bus_4_56dcc : Inport  Port=3
  State_vd_bus_5_a3b9b : Inport  Port=4
  Add_1b0ac : Sum
  Add_96d4b : Sum
  Constant_-80.0510363901558_90173 : Constant  Value=-80.0510363901558
  Constant_376.991118430775_e3072 : Constant  Value=376.991118430775
  Constant_4300.18080100745_9c7ac : Constant  Value=4300.18080100745
  Constant_4300.18080100745_a5970 : Constant  Value=4300.18080100745
  Product_0c49c : Product
  Product_9862e : Product
  Product_b8bf5 : Product
  Product_e348a : Product
  Subtract_1b9cd : Sum  Inputs=+-
  Blockout_d_id_line_4_5_7311f : Outport
  wires:
  Constant_-80.0510363901558_90173/1 -> Product_b8bf5/1
  Product_9862e/1 -> Add_96d4b/2
  State_id_line_4_5_ad13b/1 -> Product_b8bf5/2
  Constant_376.991118430775_e3072/1 -> Product_9862e/1
  State_iq_line_4_5_080ac/1 -> Product_9862e/2
  Product_b8bf5/1 -> Add_96d4b/1
  Constant_4300.18080100745_9c7ac/1 -> Product_e348a/1
  State_vd_bus_4_56dcc/1 -> Product_e348a/2
  Add_96d4b/1 -> Add_1b0ac/1
  Product_e348a/1 -> Add_1b0ac/2
  Constant_4300.18080100745_a5970/1 -> Product_0c49c/1
  State_vd_bus_5_a3b9b/1 -> Product_0c49c/2
  Add_1b0ac/1 -> Subtract_1b9cd/1
  Product_0c49c/1 -> Subtract_1b9cd/2
  Subtract_1b9cd/1 -> Blockout_d_id_line_4_5_7311f/1

== system case6/AC_1/d_id_line_5_6_block ==
  note: d_id_line_5_6 in case6
      | $376.991118430775\,\mathrm{iq}_{\mathrm{line},5,6}-99.3851621342142\,\mathrm{id}_{\mathrm{line},5,6}+2327.1566687805\,\mathrm{vd}_{\mathrm{bus},5}-2327.1566687805\,\mathrm{vd}_{\mathrm{bus},6}$
      | Automatically generated on 2025-10-31 19:20:53 .
  State_id_line_5_6_ede96 : Inport
  State_iq_line_5_6_03448 : Inport  Port=2
  State_vd_bus_5_0485d : Inport  Port=3
  State_vd_bus_6_2762e : Inport  Port=4
  Add_3b1cc : Sum
  Add_9c45f : Sum
  Constant_-99.3851621342142_edff1 : Constant  Value=-99.3851621342142
  Constant_2327.1566687805_2b091 : Constant  Value=2327.1566687805
  Constant_2327.1566687805_6fc53 : Constant  Value=2327.1566687805
  Constant_376.991118430775_ad9f6 : Constant  Value=376.991118430775
  Product_41c27 : Product
  Product_42d12 : Product
  Product_4526e : Product
  Product_c206b : Product
  Subtract_a328b : Sum  Inputs=+-
  Blockout_d_id_line_5_6_154da : Outport
  wires:
  Constant_-99.3851621342142_edff1/1 -> Product_c206b/1
  Product_41c27/1 -> Add_9c45f/2
  State_id_line_5_6_ede96/1 -> Product_c206b/2
  Constant_376.991118430775_ad9f6/1 -> Product_41c27/1
  Product_c206b/1 -> Add_9c45f/1
  State_iq_line_5_6_03448/1 -> Product_41c27/2
  Constant_2327.1566687805_6fc53/1 -> Product_42d12/1
  Product_4526e/1 -> Subtract_a328b/2
  State_vd_bus_5_0485d/1 -> Product_42d12/2
  Add_9c45f/1 -> Add_3b1cc/1
  Product_42d12/1 -> Add_3b1cc/2
  Constant_2327.1566687805_2b091/1 -> Product_4526e/1
  State_vd_bus_6_2762e/1 -> Product_4526e/2
  Add_3b1cc/1 -> Subtract_a328b/1
  Subtract_a328b/1 -> Blockout_d_id_line_5_6_154da/1

== system case6/AC_1/d_id_line_6_7_block ==
  note: d_id_line_6_7 in case6
      | $376.991118430775\,\mathrm{iq}_{\mathrm{line},6,7}-51.1437176937107\,\mathrm{id}_{\mathrm{line},6,7}+3924.76819139569\,\mathrm{vd}_{\mathrm{bus},6}-3924.76819139569\,\mathrm{vd}_{\mathrm{bus},7}$
      | Automatically generated on 2025-10-31 19:21:00 .
  State_id_line_6_7_65cd6 : Inport
  State_iq_line_6_7_b77b9 : Inport  Port=2
  State_vd_bus_6_0c641 : Inport  Port=3
  State_vd_bus_7_d448e : Inport  Port=4
  Add_375ba : Sum
  Add_f2313 : Sum
  Constant_-51.1437176937107_a9fb4 : Constant  Value=-51.1437176937107
  Constant_376.991118430775_ecfc1 : Constant  Value=376.991118430775
  Constant_3924.76819139569_214a5 : Constant  Value=3924.76819139569
  Constant_3924.76819139569_7d40a : Constant  Value=3924.76819139569
  Product_90c03 : Product
  Product_95d70 : Product
  Product_d13e8 : Product
  Product_e786d : Product
  Subtract_fb6f8 : Sum  Inputs=+-
  Blockout_d_id_line_6_7_71267 : Outport
  wires:
  Constant_-51.1437176937107_a9fb4/1 -> Product_e786d/1
  Product_d13e8/1 -> Add_375ba/2
  State_id_line_6_7_65cd6/1 -> Product_e786d/2
  Constant_376.991118430775_ecfc1/1 -> Product_d13e8/1
  State_iq_line_6_7_b77b9/1 -> Product_d13e8/2
  Product_e786d/1 -> Add_375ba/1
  Constant_3924.76819139569_214a5/1 -> Product_95d70/1
  State_vd_bus_6_0c641/1 -> Product_95d70/2
  Add_375ba/1 -> Add_f2313/1
  Product_95d70/1 -> Add_f2313/2
  Constant_3924.76819139569_7d40a/1 -> Product_90c03/1
  State_vd_bus_7_d448e/1 -> Product_90c03/2
  Add_f2313/1 -> Subtract_fb6f8/1
  Product_90c03/1 -> Subtract_fb6f8/2
  Subtract_fb6f8/1 -> Blockout_d_id_line_6_7_71267/1

== system case6/AC_1/d_id_line_7_8_block ==
  note: d_id_line_7_8 in case6
      | $376.991118430775\,\mathrm{iq}_{\mathrm{line},7,8}-51.1437176937107\,\mathrm{id}_{\mathrm{line},7,8}+5494.67546795396\,\mathrm{vd}_{\mathrm{bus},7}-5494.67546795396\,\mathrm{vd}_{\mathrm{bus},8}$
      | Automatically generated on 2025-10-31 19:21:03 .
  State_id_line_7_8_178dd : Inport
  State_iq_line_7_8_a857b : Inport  Port=2
  State_vd_bus_7_a03f4 : Inport  Port=3
  State_vd_bus_8_cba40 : Inport  Port=4
  Add_0763f : Sum
  Add_8d97c : Sum
  Constant_-51.1437176937107_1e914 : Constant  Value=-51.1437176937107
  Constant_376.991118430775_0d481 : Constant  Value=376.991118430775
  Constant_5494.67546795396_31944 : Constant  Value=5494.67546795396
  Constant_5494.67546795396_67c8b : Constant  Value=5494.67546795396
  Product_88c8f : Product
  Product_c82b4 : Product
  Product_d5114 : Product
  Product_f811f : Product
  Subtract_c6905 : Sum  Inputs=+-
  Blockout_d_id_line_7_8_868fa : Outport
  wires:
  Constant_-51.1437176937107_1e914/1 -> Product_f811f/1
  Product_d5114/1 -> Add_0763f/2
  State_id_line_7_8_178dd/1 -> Product_f811f/2
  Constant_376.991118430775_0d481/1 -> Product_d5114/1
  Product_f811f/1 -> Add_0763f/1
  State_iq_line_7_8_a857b/1 -> Product_d5114/2
  Constant_5494.67546795396_31944/1 -> Product_88c8f/1
  State_vd_bus_7_a03f4/1 -> Product_88c8f/2
  Add_0763f/1 -> Add_8d97c/1
  Product_88c8f/1 -> Add_8d97c/2
  Constant_5494.67546795396_67c8b/1 -> Product_c82b4/1
  State_vd_bus_8_cba40/1 -> Product_c82b4/2
  Add_8d97c/1 -> Subtract_c6905/1
  Product_c82b4/1 -> Subtract_c6905/2
  Subtract_c6905/1 -> Blockout_d_id_line_7_8_868fa/1

== system case6/AC_1/d_id_line_8_2_block ==
  note: d_id_line_8_2 in case6
      | $376.991118430775\,\mathrm{iq}_{\mathrm{line},8,2}-6329.86613908296\,\mathrm{vd}_{\mathrm{bus},2}+6329.86613908296\,\mathrm{vd}_{\mathrm{bus},8}$
      | Automatically generated on 2025-10-31 19:21:06 .
  State_iq_line_8_2_2a77a : Inport
  State_vd_bus_2_ddd4b : Inport  Port=2
  State_vd_bus_8_6bcd4 : Inport  Port=3
  Add_d7bd2 : Sum
  Constant_376.991118430775_0b1f6 : Constant  Value=376.991118430775
  Constant_6329.86613908296_1abb9 : Constant  Value=6329.86613908296
  Constant_6329.86613908296_6555f : Constant  Value=6329.86613908296
  Product_6a992 : Product
  Product_d21a6 : Product
  Product_dcc6d : Product
  Subtract_a3831 : Sum  Inputs=+-
  Blockout_d_id_line_8_2_da1fe : Outport
  wires:
  State_vd_bus_2_ddd4b/1 -> Product_d21a6/2
  Constant_376.991118430775_0b1f6/1 -> Product_dcc6d/1
  Product_d21a6/1 -> Subtract_a3831/2
  State_iq_line_8_2_2a77a/1 -> Product_dcc6d/2
  Constant_6329.86613908296_1abb9/1 -> Product_d21a6/1
  Product_dcc6d/1 -> Subtract_a3831/1
  Constant_6329.86613908296_6555f/1 -> Product_6a992/1
  State_vd_bus_8_6bcd4/1 -> Product_6a992/2
  Subtract_a3831/1 -> Add_d7bd2/1
  Product_6a992/1 -> Add_d7bd2/2
  Add_d7bd2/1 -> Blockout_d_id_line_8_2_da1fe/1

== system case6/AC_1/d_id_line_8_9_block ==
  note: d_id_line_8_9 in case6
      | $376.991118430775\,\mathrm{iq}_{\mathrm{line},8,9}-86.1053164532769\,\mathrm{id}_{\mathrm{line},8,9}+2457.24617200426\,\mathrm{vd}_{\mathrm{bus},8}-2457.24617200426\,\mathrm{vd}_{\mathrm{bus},9}$
      | Automatically generated on 2025-10-31 19:21:09 .
  State_id_line_8_9_91b21 : Inport
  State_iq_line_8_9_fbe05 : Inport  Port=2
  State_vd_bus_8_64db1 : Inport  Port=3
  State_vd_bus_9_80f42 : Inport  Port=4
  Add_4b069 : Sum
  Add_7a7ee : Sum
  Constant_-86.1053164532769_42319 : Constant  Value=-86.1053164532769
  Constant_2457.24617200426_46bbc : Constant  Value=2457.24617200426
  Constant_2457.24617200426_c89f8 : Constant  Value=2457.24617200426
  Constant_376.991118430775_846e8 : Constant  Value=376.991118430775
  Product_73e67 : Product
  Product_8f019 : Product
  Product_98600 : Product
  Product_a7052 : Product
  Subtract_bb7e8 : Sum  Inputs=+-
  Blockout_d_id_line_8_9_b4a61 : Outport
  wires:
  Constant_-86.1053164532769_42319/1 -> Product_73e67/1
  Product_8f019/1 -> Add_4b069/2
  State_id_line_8_9_91b21/1 -> Product_73e67/2
  Constant_376.991118430775_846e8/1 -> Product_8f019/1
  State_iq_line_8_9_fbe05/1 -> Product_8f019/2
  Product_73e67/1 -> Add_4b069/1
  Constant_2457.24617200426_c89f8/1 -> Product_a7052/1
  State_vd_bus_8_64db1/1 -> Product_a7052/2
  Add_4b069/1 -> Add_7a7ee/1
  Product_a7052/1 -> Add_7a7ee/2
  Constant_2457.24617200426_46bbc/1 -> Product_98600/1
  State_vd_bus_9_80f42/1 -> Product_98600/2
  Add_7a7ee/1 -> Subtract_bb7e8/1
  Product_98600/1 -> Subtract_bb7e8/2
  Subtract_bb7e8/1 -> Blockout_d_id_line_8_9_b4a61/1

== system case6/AC_1/d_id_line_9_4_block ==
  note: d_id_line_9_4 in case6
      | $376.991118430775\,\mathrm{iq}_{\mathrm{line},9,4}-50.9667498124176\,\mathrm{id}_{\mathrm{line},9,4}-4654.313337561\,\mathrm{vd}_{\mathrm{bus},4}+4654.313337561\,\mathrm{vd}_{\mathrm{bus},9}$
      | Automatically generated on 2025-10-31 19:21:12 .
  State_id_line_9_4_0416a : Inport
  State_iq_line_9_4_a6420 : Inport  Port=2
  State_vd_bus_4_54ca0 : Inport  Port=3
  State_vd_bus_9_b5f80 : Inport  Port=4
  Add_74b57 : Sum
  Add_b3ea0 : Sum
  Constant_-50.9667498124176_113d6 : Constant  Value=-50.9667498124176
  Constant_376.991118430775_daf68 : Constant  Value=376.991118430775
  Constant_4654.313337561_527ab : Constant  Value=4654.313337561
  Constant_4654.313337561_d70df : Constant  Value=4654.313337561
  Product_5f226 : Product
  Product_831f1 : Product
  Product_8df2b : Product
  Product_8fc5d : Product
  Subtract_51f6b : Sum  Inputs=+-
  Blockout_d_id_line_9_4_cfcaf : Outport
  wires:
  Constant_-50.9667498124176_113d6/1 -> Product_5f226/1
  Product_8fc5d/1 -> Add_74b57/2
  State_id_line_9_4_0416a/1 -> Product_5f226/2
  Constant_376.991118430775_daf68/1 -> Product_8fc5d/1
  Product_5f226/1 -> Add_74b57/1
  State_iq_line_9_4_a6420/1 -> Product_8fc5d/2
  Constant_4654.313337561_527ab/1 -> Product_831f1/1
  State_vd_bus_4_54ca0/1 -> Product_831f1/2
  Add_74b57/1 -> Subtract_51f6b/1
  Product_831f1/1 -> Subtract_51f6b/2
  Constant_4654.313337561_d70df/1 -> Product_8df2b/1
  Subtract_51f6b/1 -> Add_b3ea0/1
  State_vd_bus_9_b5f80/1 -> Product_8df2b/2
  Product_8df2b/1 -> Add_b3ea0/2
  Add_b3ea0/1 -> Blockout_d_id_line_9_4_cfcaf/1

== system case6/AC_1/d_id_load_5_block ==
  note: d_id_load_5 in case6
      | $376.991118430775\,\mathrm{iq}_{\mathrm{load},5}-1094.814270933\,\mathrm{id}_{\mathrm{load},5}+1121.6545740232\,\mathrm{vd}_{\mathrm{bus},5}$
      | Automatically generated on 2025-10-31 19:20:38 .
  State_id_load_5_13a8a : Inport
  State_iq_load_5_cadf3 : Inport  Port=2
  State_vd_bus_5_d8d97 : Inport  Port=3
  Add_5fba8 : Sum
  Add_bf8c4 : Sum
  Constant_-1094.814270933_f4739 : Constant  Value=-1094.814270933
  Constant_1121.6545740232_68b7b : Constant  Value=1121.6545740232
  Constant_376.991118430775_11d41 : Constant  Value=376.991118430775
  Product_525d2 : Product
  Product_6da8b : Product
  Product_b4f90 : Product
  Blockout_d_id_load_5_e47ee : Outport
  wires:
  Constant_-1094.814270933_f4739/1 -> Product_6da8b/1
  Product_b4f90/1 -> Add_bf8c4/2
  State_id_load_5_13a8a/1 -> Product_6da8b/2
  Constant_376.991118430775_11d41/1 -> Product_b4f90/1
  Product_525d2/1 -> Add_5fba8/2
  State_iq_load_5_cadf3/1 -> Product_b4f90/2
  Product_6da8b/1 -> Add_bf8c4/1
  Constant_1121.6545740232_68b7b/1 -> Product_525d2/1
  State_vd_bus_5_d8d97/1 -> Product_525d2/2
  Add_bf8c4/1 -> Add_5fba8/1
  Add_5fba8/1 -> Blockout_d_id_load_5_e47ee/1
